simulink model "hw2_eserc_5_simulink_integrator"  (R2023b)
settings: Solver=FixedStepDiscrete  StartTime=0.0  StopTime=3.0  FixedStep=0.01  RelTol=1e-3
settings Model: Creator=lalla  LastModifiedBy=lalla

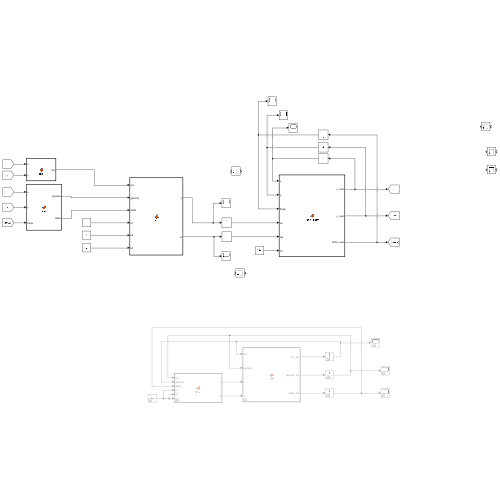
[thumbnail: Simulink's stored preview of the top-level diagram]
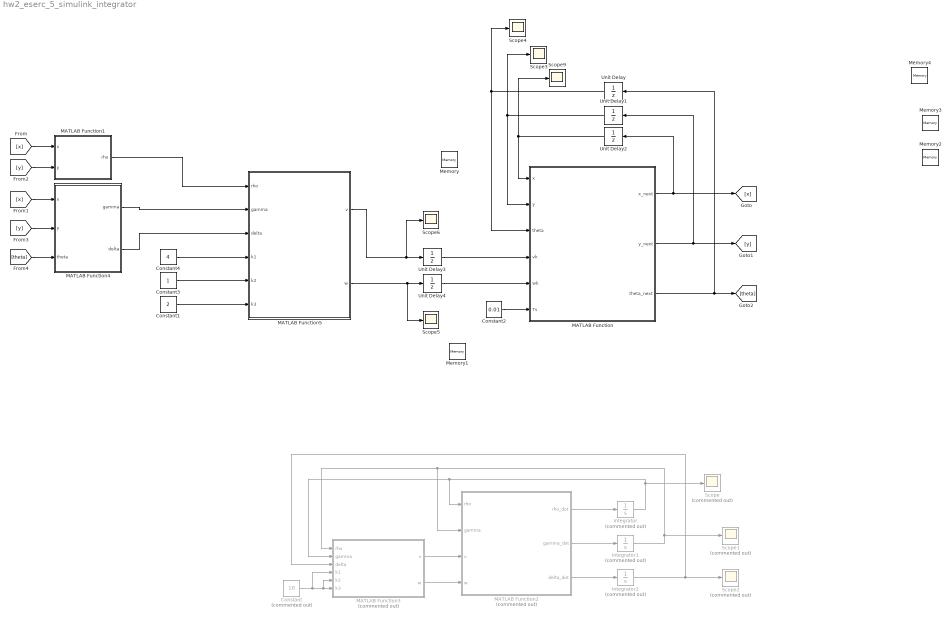
== system hw2_eserc_5_simulink_integrator ==
  Constant : Constant  Commented=on  Value=10
  Constant1 : Constant  Value=2
  Constant2 : Constant  Value=0.01
  Constant3 : Constant
  Constant4 : Constant  Value=4
  Integrator : Integrator  Commented=on  InitialCondition=10
  Integrator1 : Integrator  Commented=on  InitialCondition=pi
  Integrator2 : Integrator  Commented=on
  MATLAB Function : MATLAB Function  Tag=inte  TreatAsAtomicUnit=on
  MATLAB Function1 : MATLAB Function  TreatAsAtomicUnit=on
  MATLAB Function2 : MATLAB Function  Commented=on  TreatAsAtomicUnit=on
  MATLAB Function3 : MATLAB Function  Commented=on  TreatAsAtomicUnit=on
  MATLAB Function4 : MATLAB Function  TreatAsAtomicUnit=on
  MATLAB Function5 : MATLAB Function  TreatAsAtomicUnit=on
  Memory : Memory
  Memory1 : Memory
  Memory2 : Memory  InitialCondition=1
  Memory3 : Memory  InitialCondition=1
  Memory4 : Memory  InitialCondition=pi/4
  Scope : Scope  Commented=on
  Scope1 : Scope  Commented=on
  Scope2 : Scope  Commented=on
  Scope{3..6,9} (5 alike) : Scope
  Unit Delay : UnitDelay  InitialCondition=pi/4  SampleTime=-1  HasFrameUpgradeWarning=on
  Unit Delay1 : UnitDelay  InitialCondition=1  SampleTime=-1  HasFrameUpgradeWarning=on
  Unit Delay2 : UnitDelay  InitialCondition=1  SampleTime=-1  HasFrameUpgradeWarning=on
  Unit Delay3 : UnitDelay  SampleTime=-1  HasFrameUpgradeWarning=on
  Unit Delay4 : UnitDelay  SampleTime=-1  HasFrameUpgradeWarning=on
  wires:
  MATLAB Function/1(x_next) -> Unit Delay2/1, [x]
  MATLAB Function/2(y_next) -> Unit Delay1/1, [y]
  MATLAB Function2/3(delta_dot) -> Integrator2/1
  MATLAB Function2/2(gamma_dot) -> Integrator1/1
  MATLAB Function2/1(rho_dot) -> Integrator/1
  Integrator2/1 -> Scope2/1, MATLAB Function3/3(delta)
  Integrator/1 -> Scope/1, MATLAB Function3/2(gamma), MATLAB Function2/1(rho)
  Integrator1/1 -> Scope1/1, MATLAB Function3/1(rho), MATLAB Function2/2(gamma)
  MATLAB Function3/1(v) -> MATLAB Function2/3(v)
  MATLAB Function3/2(w) -> MATLAB Function2/4(w)
  Constant/1 -> MATLAB Function3/4(k1), MATLAB Function3/5(k2), MATLAB Function3/6(k3)
  MATLAB Function/3(theta_next) -> Unit Delay/1, [theta]
  MATLAB Function4/1(gamma) -> MATLAB Function5/2(gamma)
  MATLAB Function1/1(rho) -> MATLAB Function5/1(rho)
  MATLAB Function4/2(delta) -> MATLAB Function5/3(delta)
  Constant1/1 -> MATLAB Function5/6(k3)
  MATLAB Function5/2(w) -> Unit Delay4/1, Scope5/1
  MATLAB Function5/1(v) -> Unit Delay3/1, Scope6/1
  Unit Delay/1 -> Scope4/1, MATLAB Function/3(theta)
  Unit Delay1/1 -> Scope3/1, MATLAB Function/2(y)
  Unit Delay2/1 -> Scope9/1, MATLAB Function/1(x)
  Unit Delay4/1 -> MATLAB Function/5(wk)
  Unit Delay3/1 -> MATLAB Function/4(vk)
  Constant2/1 -> MATLAB Function/6(Ts)
  [x] -> MATLAB Function1/1(x)
  [x] -> MATLAB Function4/1(x)
  [y] -> MATLAB Function1/2(y)
  [y] -> MATLAB Function4/2(y)
  [theta] -> MATLAB Function4/3(theta)
  Constant3/1 -> MATLAB Function5/5(k2)
  Constant4/1 -> MATLAB Function5/4(k1)

== matlab function hw2_eserc_5_simulink_integrator/MATLAB Function1 ==
  data: x input; rho output; y input
function rho = fcn(x,y)
rho = sqrt(x^2 + y^2);

== matlab function hw2_eserc_5_simulink_integrator/MATLAB Function ==
  data: x input; x_next output; y input; theta input; vk input; wk input; Ts input; y_next output; theta_next output
function [x_next,y_next,theta_next] = Ruge_kutta(x,y,theta,vk,wk,Ts)
x_next = x +vk*Ts*cos(theta+wk*Ts/2);
y_next = y +vk*Ts*sin(theta+wk*Ts/2);
theta_next = theta + wk*Ts;

== matlab function hw2_eserc_5_simulink_integrator/MATLAB Function2 ==
  data: rho input; rho_dot output; gamma input; v input; w input; gamma_dot output; delta_dot output
function [rho_dot, gamma_dot, delta_dot] = fcn(rho,gamma,v,w)
rho_dot = -v*cos(gamma);
gamma_dot = sin(gamma)*v/rho - w;
delta_dot = sin(gamma)*v/rho;

== matlab function hw2_eserc_5_simulink_integrator/MATLAB Function3 ==
  data: rho input; v output; gamma input; delta input; k1 input; k2 input; k3 input; w output
function [v,w] = fcn(rho,gamma,delta,k1,k2,k3)
v=k1*rho*cos(gamma);
w=k2*gamma+k1*sin(gamma)*cos(gamma)*(1+k3*delta/gamma);

== matlab function hw2_eserc_5_simulink_integrator/MATLAB Function4 ==
  data: x input; gamma output; y input; theta input; delta output
function [gamma,delta] = fcn(x,y,theta)
gamma = atan2(y,x) - theta + pi;
delta = atan2(y,x) + pi;

== matlab function hw2_eserc_5_simulink_integrator/MATLAB Function5 ==
  data: rho input; v output; gamma input; delta input; k1 input; k2 input; k3 input; w output
function [v,w] = fcn(rho,gamma,delta,k1,k2,k3)
v=k1*rho*cos(gamma);
w=k2*gamma+k1*sin(gamma)*cos(gamma)*(1+k3*delta/gamma);
